simulink model "B2"  (R2023a)
settings: Solver=VariableStepAuto  StartTime=0.0  StopTime=10  RelTol=1e-3
undefined symbols (not defined in the file): K, L, omega
settings Model: Creator=86173  LastModifiedBy=86173

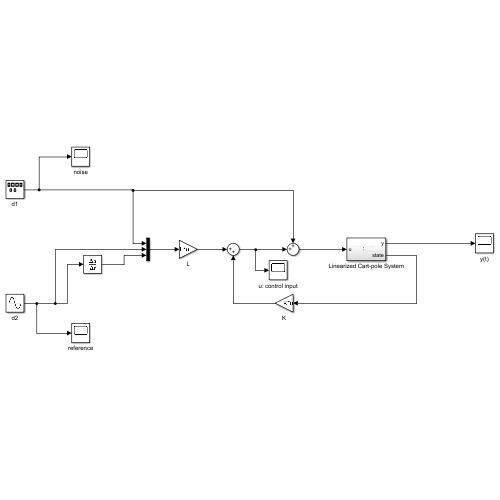
[thumbnail: Simulink's stored preview of the top-level diagram]
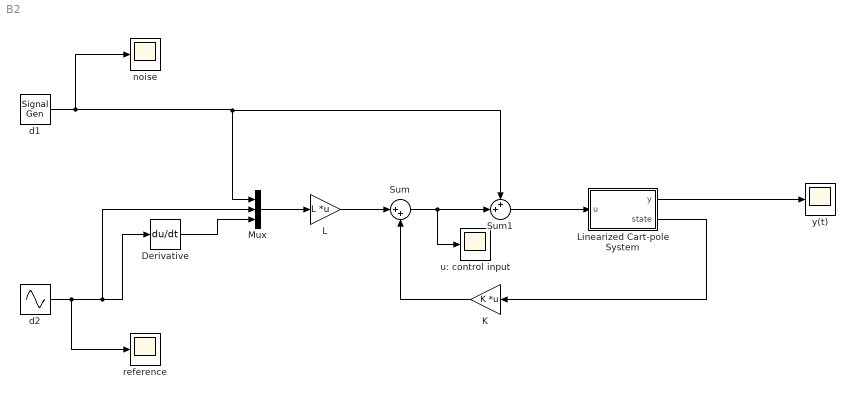
== system B2 ==
  Derivative : Derivative
  K : Gain  Gain=K  Multiplication=Matrix(K*u)
  L : Gain  Gain=L  Multiplication=Matrix(K*u)
  Linearized Cart-pole System : Subsystem
  Mux : Mux  Inputs=3
  Sum : Sum  Inputs=|++
  Sum1 : Sum  Inputs=++|
  d1 : SignalGenerator  WaveForm=square  Amplitude=0.5  Frequency=0.02
  d2 : Sin  Frequency=omega  SampleTime=0
  noise : Scope
  reference : Scope
  u: control input : Scope
  y(t) : Scope
  wires:
  Linearized Cart-pole System/2(state) -> K/1
  Mux/1 -> L/1
  d2/1 -> reference/1, Derivative/1, Mux/2
  Derivative/1 -> Mux/3
  K/1 -> Sum/2
  L/1 -> Sum/1
  d1/1 -> noise/1, Sum1/1, Mux/1
  Sum1/1 -> Linearized Cart-pole System/1(u)
  Sum/1 -> u: control input/1, Sum1/2
  Linearized Cart-pole System/1(y) -> y(t)/1

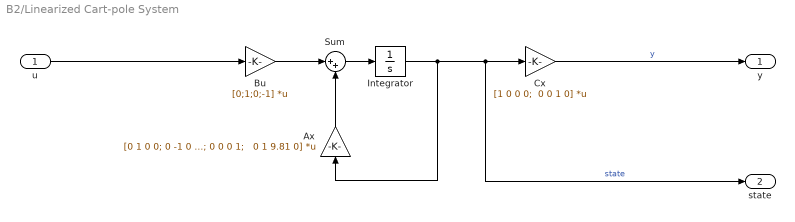
== system B2/Linearized Cart-pole System ==
  u : Inport
  Ax : Gain  Gain=|  Multiplication=Matrix(K*u)
      | [0 1 0 0;
      | 0 -1 0 0;
      | 0 0 0 1;
      |   0 1 9.81 0]
  Bu : Gain  Gain=[0;1;0;-1]  Multiplication=Matrix(K*u)
  Cx : Gain  Gain=|  Multiplication=Matrix(K*u)
      | [1 0 0 0;
      |  0 0 1 0]
  Integrator : Integrator
  Sum : Sum  Inputs=|++
  y : Outport
  state : Outport  Port=2
  wires:
  Cx/1 -> y/1  "y"
  Integrator/1 -> Ax/1, state/1, Cx/1  "state"
  Bu/1 -> Sum/1
  Ax/1 -> Sum/2
  u/1 -> Bu/1
  Sum/1 -> Integrator/1
